simulink model "Waarnemer"  (R2020b)
settings: Solver=VariableStepAuto  StartTime=0.0  StopTime=10.0  RelTol=1e-3
libraries: powerlib x11
settings Model: Creator=Tijl J  LastModifiedBy=Tijl J

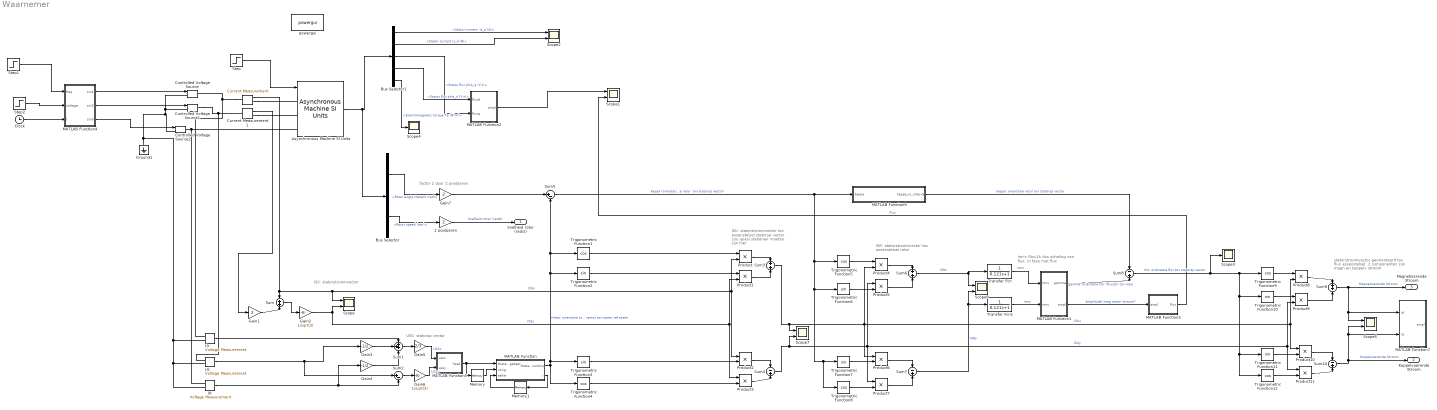
== system Waarnemer ==
  note: Imr= flux/Lh dus schaling
      | van flux, in fase met flux
  note: factor 2 door 2 poolparen
  note: statorstroomvector georienteerd
      | tov flux assenstelsel: 2 componenten
      | zijn magn en koppelv stroom
  note: ISS: statorstroomvector
  note: USS: statorsp vector
  note: ISR: statorstroomvector tov
      | assenstelsel rotor
  note: ISU: statorstroomvector tov
      | assenstelsel statorsp vector
      | zou quasi stationair moeten
      | zijn hier
  " " : powerlib/Measurements/Current Measurement  PhasorSimulation=off  OutputType=Complex  PSBequivalent=0
  2 poolparen : Gain  Gain=2
  Asynchronous Machine SI Units : powerlib/Machines/Asynchronous Machine SI Units  RotorType=Squirrel-cage  PresetModel="15:  5.4 HP (4KW)   400 V  50Hz 1430 RPM"  MechanicalLoad=Torque Tm  ShowDetailedParameters=on  ReferenceFrame=Synchronous  Units=SI  MeasurementBus=off  NominalParameters=[4000 400 50]  Stator=[1.405 0.005839]  Rotor=[1.395 0.005839]  Cage1=[0.4155 0.002066]  Cage2=[0.4168 0.0003495]  Lm=0.1722  Mechanical=[0.0131 0.002985 2]  PolePairs=2  InitialConditions=[0 0 0 0 0 0 0 0]  SimulateSaturation=off  Saturation=[14.03593122, 27.81365428, 53.79336849, 68, 82, 96, 110,124, 130 ; 230, 322, 414, 460, 506, 552, 598, 644, 690]  LoadFlowParameters=1492000  TsPowergui=0  TsBlock=-1  IterativeModel=Trapezoidal non iterative  IterativeDiscreteModel=Trapezoidal non iterative  Pmec=1.492e+006
  Bus Selector : BusSelector  OutputSignals=Mechanical.Rotor angle thetam (rad),Mechanical.Rotor speed (wm)
  Bus Selector1 : BusSelector  OutputSignals="Stator measurements.Stator current  is_q (A),Stator measurements.Stator current is_d (A),Stator measurements.Stator flux phis_q (V s),Stator measurements.Stator flux phis_d (V s),Mechanical.Electromagnetic torque Te (N*m)"
  Clock : Clock
  Controlled Voltage Source : powerlib/Electrical Sources/Controlled Voltage Source  Initialize=on  Source_Type=AC  Amplitude=0  Phase=0  Frequency=0  Measurements=None
  Controlled Voltage Source1 : powerlib/Electrical Sources/Controlled Voltage Source  Initialize=on  Source_Type=AC  Amplitude=0  Phase=0  Frequency=0  Measurements=None
  Controlled Voltage Source2 : powerlib/Electrical Sources/Controlled Voltage Source  Initialize=on  Source_Type=AC  Amplitude=0  Phase=0  Frequency=0  Measurements=None
  Current Measurement1 : powerlib/Measurements/Current Measurement  PhasorSimulation=off  OutputType=Complex  PSBequivalent=0
  Gain1 : Gain  Gain=2
  Gain2 : Gain  Gain=1/sqrt(3)
  Gain3 : Gain  Gain=-1/2
  Gain4 : Gain  Gain=-1/2
  Gain5 : Gain  Gain=2/3
  Gain6 : Gain  Gain=1/sqrt(3)
  Gain7 : Gain  Gain=2
  Ground1 : powerlib/Elements/Ground  LConnTagsString=a
  MATLAB Function : MATLAB Function  TreatAsAtomicUnit=on
  MATLAB Function1 : MATLAB Function  TreatAsAtomicUnit=on
  MATLAB Function2 : MATLAB Function  TreatAsAtomicUnit=on
  MATLAB Function3 : MATLAB Function  TreatAsAtomicUnit=on
  MATLAB Function4 : MATLAB Function  TreatAsAtomicUnit=on
  MATLAB Function5 : MATLAB Function  TreatAsAtomicUnit=on
  MATLAB Function7 : MATLAB Function  TreatAsAtomicUnit=on
  MATLAB Function9 : MATLAB Function  TreatAsAtomicUnit=on
  Memory : Memory
  Memory1 : Memory
  Product{,1..11} (12 alike) : Product
  Scope{,1..2,5,7..8} (6 alike) : Scope  NumInputPorts=2
  Scope3 : Scope
  Scope4 : Scope
  Step : Step  Time=0  After=0  SampleTime=0
  Step1 : Step  Time=0  After=50  SampleTime=0
  Step2 : Step  Time=0  After=326  SampleTime=0
  Sum : Sum
  Sum1 : Sum  Inputs=3
  Sum{4,7..8,10} (4 alike) : Sum  Inputs=-+
  Sum2 : Sum  Inputs=|+-
  Sum3 : Sum  Inputs=2
  Sum5 : Sum  Inputs=|+-
  Sum6 : Sum
  Sum9 : Sum
  Transfer Fcn : TransferFcn  Denominator=[0.121 1]
  Transfer Fcn1 : TransferFcn  Denominator=[0.121 1]
  Trigonometric Function{1,4..5,8..9,12} (6 alike) : Trigonometry  Operator=cos
  Trigonometric Function{2..3,6..7,10..11} (6 alike) : Trigonometry
  Ur : powerlib/Measurements/Voltage Measurement  PhasorSimulation=off  OutputType=Complex  PSBequivalent=0
  Us : powerlib/Measurements/Voltage Measurement  PhasorSimulation=off  OutputType=Complex  PSBequivalent=0
  Ut : powerlib/Measurements/Voltage Measurement  PhasorSimulation=off  OutputType=Complex  PSBequivalent=0
  powergui : powerlib/powergui  Priority=1  SimulationMode=Continuous  SampleTime=50e-6  frequency=60  Iterations=50  frequencyindice=50  Pbase=100e6  ErrMax=1e-4  UnitsV=kV  UnitsW=MW  buscounter=0  FunctionMessages=off  echomessages=off  EnableUseOfTLC=off  CurrentSourceSwitches=off  DisableSnubberDevices=off  DisableRonSwitches=off  DisableVfSwitches=off  DisplayEquations=off  AutomaticDiscreteSolvers=off  SolverType=Tustin/Backward Euler (TBE)  Interpol=off  ExternalGateDelay=off  methode=off  Ts=100  x0status=blocks  SPID=on  SwTol=0  HookPort=off  NonlinearTolerance=1e-4  nMaxIteration=100  ContinueOnMaxIteration=off  RestoreLinks=warning  ResistiveCurrentMeasurement=off  Frange=[0:2:500]  Ylog=off  Xlog=on  ShowGrid=off  save=off  variable=ZData  structure=0  ZoomFFT=off  StartTime=0.0  cycles=1  DisplayStyle=1  fundamental=60  FreqAxis=off  MaxFrequency=1000  frequencyindicesteady=1  RmsSteady=1  display=off
  Snelheid rotor (rad/s) : Outport
  Koppelvoerende Stroom : Outport  Port=2
  Magnetiserende Stroom : Outport  Port=3
  wires:
  Bus Selector1/1 -> Scope2/1  "<Stator current  is_q (A)>"
  Bus Selector1/2 -> Scope2/2  "<Stator current is_d (A)>"
  Step/1 -> Asynchronous Machine SI Units/1
  MATLAB Function4/2(sin2) -> Controlled Voltage Source1/1
  MATLAB Function4/3(sin3) -> Controlled Voltage Source2/1
  Clock/1 -> MATLAB Function4/3(t)
  Step1/1 -> MATLAB Function4/1(freq)
  MATLAB Function4/1(sin1) -> Controlled Voltage Source/1
  Step2/1 -> MATLAB Function4/2(voltage)
  Us/1 -> Gain3/1, Sum2/1
  Asynchronous Machine SI Units/1 -> Bus Selector/1, Bus Selector1/1
  MATLAB Function/1(theta_continu) -> Trigonometric Function1/1, Sum5/2, Trigonometric Function2/1, Trigonometric Function3/1, Trigonometric Function4/1  "theta: orientatie stator sp vector tov stator ref assen"
  Sum4/1 -> Scope7/2, Product5/1, Product9/2, Product11/1, Product7/1  "ISUy"
  Trigonometric Function8/1 -> Product7/2
  Gain1/1 -> Sum/2
  Bus Selector/1 -> Gain7/1  "<Rotor angle thetam (rad)>"
  Memory/1 -> MATLAB Function/2(vorig)
  Product6/1 -> Sum7/1
  Gain2/1 -> Scope/2, Product1/2, Product3/1  "ISSy"
  Trigonometric Function9/1 -> Product8/1
  " "/1 -> Sum/1, Scope/1, Product/2, Product2/1  "ISSx"
  Trigonometric Function6/1 -> Product5/2
  Sum6/1 -> Transfer Fcn/1, Scope8/1  "ISRx"
  Trigonometric Function7/1 -> Product6/2
  MATLAB Function1/2(ampl) -> MATLAB Function3/1(ampl)  "Amplitude imag stator stroom?"
  2 poolparen/1 -> Snelheid rotor (rad/s)/1  "Snelheid rotor (rad/s)"
  Product1/1 -> Sum3/2
  Product4/1 -> Sum6/1
  Product5/1 -> Sum6/2
  Sum9/1 -> Scope5/1, MATLAB Function7/1(id), Magnetiserende Stroom/1  "Magnetiserende Stroom"
  Sum2/1 -> Gain6/1
  Sum/1 -> Gain2/1
  Sum10/1 -> Koppelvoerende Stroom/1, Scope5/2, MATLAB Function7/2(iq)  "Koppelvoerende Stroom"
  Sum5/1 -> MATLAB Function9/1(kappa), Trigonometric Function7/1, Trigonometric Function8/1, Trigonometric Function6/1, Trigonometric Function5/1  "kappa (orientatie rotor  tov statorsp vector)"
  MATLAB Function5/1(hoek) -> MATLAB Function/1(theta_gekapt), Memory/1
  Current Measurement1/1 -> Gain1/1
  Trigonometric Function11/1 -> Product10/2
  MATLAB Function9/1(kappa_in_interval) -> Sum8/1  "kappa: orientatie rotor tov statorsp vector"
  Gain5/1 -> MATLAB Function5/1(ussx)  "USSx"
  Transfer Fcn/1 -> MATLAB Function1/1(imrx)  "Imrx"
  Memory1/1 -> MATLAB Function/3(teller)
  Trigonometric Function3/1 -> Product2/2
  MATLAB Function3/1(flux) -> Scope1/2  "Flux"
  MATLAB Function1/1(gamma) -> Sum8/2  "gamma: oriëntatie Imr (flux/Lh) tov rotor"
  Trigonometric Function4/1 -> Product3/2
  Product10/1 -> Sum10/1
  Gain7/1 -> Sum5/1
  Trigonometric Function2/1 -> Product1/1
  Trigonometric Function10/1 -> Product9/1
  Gain4/1 -> Sum1/3
  Trigonometric Function12/1 -> Product11/2
  Gain3/1 -> Sum1/2
  Ut/1 -> Gain4/1, Sum2/2
  Product8/1 -> Sum9/1
  Ur/1 -> Sum1/1
  Sum8/1 -> Scope3/1, Trigonometric Function12/1, Trigonometric Function11/1, Trigonometric Function10/1, Trigonometric Function9/1  "rho: oriëntatie flux tov statorsp vector"
  Sum7/1 -> Scope8/2, Transfer Fcn1/1  "ISRy"
  Product2/1 -> Sum4/1
  Product11/1 -> Sum10/2
  Product7/1 -> Sum7/2
  Bus Selector/2 -> 2 poolparen/1  "<Rotor speed (wm)>"
  Trigonometric Function5/1 -> Product4/1
  Gain6/1 -> MATLAB Function5/2(ussy)  "USSy"
  MATLAB Function/2(i) -> Memory1/1
  Product/1 -> Sum3/1
  Product9/1 -> Sum9/2
  Trigonometric Function1/1 -> Product/1
  Transfer Fcn1/1 -> MATLAB Function1/2(imry)  "Imry"
  Sum1/1 -> Gain5/1
  Product3/1 -> Sum4/2
  Sum3/1 -> Scope7/1, Product4/2, Product8/2, Product10/1, Product6/1  "ISUx"
  MATLAB Function2/1(ampl) -> Scope1/1
  Bus Selector1/3 -> MATLAB Function2/2(fluxq)  "<Stator flux phis_q (V s)>"
  Bus Selector1/4 -> MATLAB Function2/1(fluxd)  "<Stator flux phis_d (V s)>"
  Bus Selector1/5 -> Scope4/1  "<Electromagnetic torque Te (N*m)>"
  connections:
  Us/LConn2 -- Ur/LConn2 -- Controlled Voltage Source2/LConn1 -- Controlled Voltage Source1/LConn1 -- Controlled Voltage Source/LConn1 -- Ground1/LConn1 -- Ut/LConn2
  Controlled Voltage Source2/RConn1 -- Ut/LConn1 -- Asynchronous Machine SI Units/LConn3
  " "/LConn1 -- Controlled Voltage Source/RConn1 -- Ur/LConn1
  Current Measurement1/RConn1 -- Asynchronous Machine SI Units/LConn2
  " "/RConn1 -- Asynchronous Machine SI Units/LConn1
  Controlled Voltage Source1/RConn1 -- Us/LConn1 -- Current Measurement1/LConn1

== matlab function Waarnemer/MATLAB Function1 ==
  data: gamma output; imrx input; ampl output; imry input
function [gamma,ampl] = fcn(imrx,imry)
ampl = sqrt(imrx^2+imry^2);
gamma = atan2(imry,imrx); %% geeft radialen weer
end

== matlab function Waarnemer/MATLAB Function ==
  data: theta_gekapt input; theta_continu output; vorig input; teller input; i output
function [theta_continu,i] = fcn(theta_gekapt,vorig,teller)
i=teller;
if isempty(vorig)
   theta_continu=theta_gekapt ;
else
    if theta_gekapt<0 && vorig>0
        i=teller+1;
    end
    theta_continu=theta_gekapt+i*2*pi;    
end
end

== matlab function Waarnemer/MATLAB Function2 ==
  data: fluxd input; ampl output; fluxq input
function ampl  = fcn(fluxd,fluxq)
ampl = sqrt(fluxd^2+fluxq^2);
end

== matlab function Waarnemer/MATLAB Function3 ==
  data: ampl input; flux output
function flux = fcn(ampl)

flux = 0.1722 * ampl; % met verzadiging wordt deze formule ingewikkelder

== matlab function Waarnemer/MATLAB Function4 ==
  data: freq input; sin1 output; voltage input; t input; sin2 output; sin3 output
function [sin1, sin2, sin3] = fcn(freq,voltage,t)

sin1 = voltage * sin(2*pi*freq*t);
sin2 = voltage * sin(2*pi*freq*t-2*pi/3);
sin3 = voltage * sin(2*pi*freq*t-4*pi/3);



end

== matlab function Waarnemer/MATLAB Function5 ==
  data: ussx input; hoek output; ussy input
function hoek = fcn(ussx,ussy)

hoek = atan2(ussy,ussx);
end

== matlab function Waarnemer/MATLAB Function7 ==
  data: id input; ampl output; iq input
function ampl  = fcn(id,iq)
ampl = sqrt(id^2+iq^2);
end

== matlab function Waarnemer/MATLAB Function9 ==
  data: kappa input; kappa_in_interval output
function kappa_in_interval = fcn(kappa)
if kappa> -pi &&kappa<pi
    kappa_in_interval=-kappa;
    
else

    kappa_in_interval=-(mod(kappa-pi,2*pi)-pi);

end
end
